simulink model "UberSpurs_oneSpur"  (R2015b)
settings: Solver=VariableStepAuto  StartTime=0.0  StopTime=5000  RelTol=1e-3
libraries: simulink x18
(part 2 of 2)

== system UberSpurs_oneSpur/spur1WorkCell/route2Channel2 ==
  serverAvailable : Inport
  Constant : Constant  Value=2
  Get Attribute : GetAttribute  AttributeName=Channel  EvaluatedDefaultAttributeValue={ []}
      settings: OutputPortMap=o1
  RoutingControlActuator : OutputSwitch  NumberOutputPorts=2  SwitchingCriterion=From signal port p  InitialConditionsOpt=on
  RoutingControlBehavior : Stateflow chart  TreatAsAtomicUnit=on
  Single Server1 : SingleServer  ServiceTime=0
  toChannel : PMIOPort  Port=1  Side=Right
  fromMHS : PMIOPort  Port=2  Side=Left
  toMHS : PMIOPort  Port=3  Side=Right
  wires:
  RoutingControlBehavior/1(route) -> RoutingControlActuator/1
  Constant/1 -> RoutingControlBehavior/2(channel)
  Get Attribute/1 -> RoutingControlBehavior/1(entityChannel)
  serverAvailable/1 -> RoutingControlBehavior/3(serverAvailable)
  connections:
  RoutingControlActuator/RConn2 -- toMHS/RConn1
  Get Attribute/RConn1 -- Single Server1/LConn1
  fromMHS/RConn1 -- Get Attribute/LConn1
  toChannel/RConn1 -- RoutingControlActuator/RConn1
  Single Server1/RConn1 -- RoutingControlActuator/LConn1

== system UberSpurs_oneSpur/spur1WorkCell/route2Channel3 ==
  serverAvailable : Inport
  Constant : Constant  Value=3
  Get Attribute : GetAttribute  AttributeName=Channel  EvaluatedDefaultAttributeValue={ []}
      settings: OutputPortMap=o1
  RoutingControlActuator : OutputSwitch  NumberOutputPorts=2  SwitchingCriterion=From signal port p  InitialConditionsOpt=on
  RoutingControlBehavior : Stateflow chart  TreatAsAtomicUnit=on
  Single Server1 : SingleServer  ServiceTime=0
  toChannel : PMIOPort  Port=1  Side=Right
  fromMHS : PMIOPort  Port=2  Side=Left
  toMHS : PMIOPort  Port=3  Side=Right
  wires:
  RoutingControlBehavior/1(route) -> RoutingControlActuator/1
  Constant/1 -> RoutingControlBehavior/2(channel)
  Get Attribute/1 -> RoutingControlBehavior/1(entityChannel)
  serverAvailable/1 -> RoutingControlBehavior/3(serverAvailable)
  connections:
  RoutingControlActuator/RConn2 -- toMHS/RConn1
  Get Attribute/RConn1 -- Single Server1/LConn1
  fromMHS/RConn1 -- Get Attribute/LConn1
  toChannel/RConn1 -- RoutingControlActuator/RConn1
  Single Server1/RConn1 -- RoutingControlActuator/LConn1

== system UberSpurs_oneSpur/spur1WorkCell/route2Channel4 ==
  serverAvailable : Inport
  Constant : Constant  Value=4
  Get Attribute : GetAttribute  AttributeName=Channel  EvaluatedDefaultAttributeValue={ []}
      settings: OutputPortMap=o1
  RoutingControlActuator : OutputSwitch  NumberOutputPorts=2  SwitchingCriterion=From signal port p  InitialConditionsOpt=on
  RoutingControlBehavior : Stateflow chart  TreatAsAtomicUnit=on
  Single Server1 : SingleServer  ServiceTime=0
  toChannel : PMIOPort  Port=1  Side=Right
  fromMHS : PMIOPort  Port=2  Side=Left
  toMHS : PMIOPort  Port=3  Side=Right
  wires:
  RoutingControlBehavior/1(route) -> RoutingControlActuator/1
  Constant/1 -> RoutingControlBehavior/2(channel)
  Get Attribute/1 -> RoutingControlBehavior/1(entityChannel)
  serverAvailable/1 -> RoutingControlBehavior/3(serverAvailable)
  connections:
  RoutingControlActuator/RConn2 -- toMHS/RConn1
  Get Attribute/RConn1 -- Single Server1/LConn1
  fromMHS/RConn1 -- Get Attribute/LConn1
  toChannel/RConn1 -- RoutingControlActuator/RConn1
  Single Server1/RConn1 -- RoutingControlActuator/LConn1

== system UberSpurs_oneSpur/spur1WorkCell/route2Channel5 ==
  serverAvailable : Inport
  Constant : Constant  Value=5
  Get Attribute : GetAttribute  AttributeName=Channel  EvaluatedDefaultAttributeValue={ []}
      settings: OutputPortMap=o1
  RoutingControlActuator : OutputSwitch  NumberOutputPorts=2  SwitchingCriterion=From signal port p  InitialConditionsOpt=on
  RoutingControlBehavior : Stateflow chart  TreatAsAtomicUnit=on
  Single Server1 : SingleServer  ServiceTime=0
  toChannel : PMIOPort  Port=1  Side=Right
  fromMHS : PMIOPort  Port=2  Side=Left
  toMHS : PMIOPort  Port=3  Side=Right
  wires:
  RoutingControlBehavior/1(route) -> RoutingControlActuator/1
  Constant/1 -> RoutingControlBehavior/2(channel)
  Get Attribute/1 -> RoutingControlBehavior/1(entityChannel)
  serverAvailable/1 -> RoutingControlBehavior/3(serverAvailable)
  connections:
  RoutingControlActuator/RConn2 -- toMHS/RConn1
  Get Attribute/RConn1 -- Single Server1/LConn1
  fromMHS/RConn1 -- Get Attribute/LConn1
  toChannel/RConn1 -- RoutingControlActuator/RConn1
  Single Server1/RConn1 -- RoutingControlActuator/LConn1

== system UberSpurs_oneSpur/spur1WorkCell/route2Channel6 ==
  serverAvailable : Inport
  Constant : Constant  Value=6
  Get Attribute : GetAttribute  AttributeName=Channel  EvaluatedDefaultAttributeValue={ []}
      settings: OutputPortMap=o1
  RoutingControlActuator : OutputSwitch  NumberOutputPorts=2  SwitchingCriterion=From signal port p  InitialConditionsOpt=on
  RoutingControlBehavior : Stateflow chart  TreatAsAtomicUnit=on
  Single Server1 : SingleServer  ServiceTime=0
  toChannel : PMIOPort  Port=1  Side=Right
  fromMHS : PMIOPort  Port=2  Side=Left
  toMHS : PMIOPort  Port=3  Side=Right
  wires:
  RoutingControlBehavior/1(route) -> RoutingControlActuator/1
  Constant/1 -> RoutingControlBehavior/2(channel)
  Get Attribute/1 -> RoutingControlBehavior/1(entityChannel)
  serverAvailable/1 -> RoutingControlBehavior/3(serverAvailable)
  connections:
  RoutingControlActuator/RConn2 -- toMHS/RConn1
  Get Attribute/RConn1 -- Single Server1/LConn1
  fromMHS/RConn1 -- Get Attribute/LConn1
  toChannel/RConn1 -- RoutingControlActuator/RConn1
  Single Server1/RConn1 -- RoutingControlActuator/LConn1

== system UberSpurs_oneSpur/spur1WorkCell/route2Channel7 ==
  serverAvailable : Inport
  Constant : Constant  Value=7
  Get Attribute : GetAttribute  AttributeName=Channel  EvaluatedDefaultAttributeValue={ []}
      settings: OutputPortMap=o1
  RoutingControlActuator : OutputSwitch  NumberOutputPorts=2  SwitchingCriterion=From signal port p  InitialConditionsOpt=on
  RoutingControlBehavior : Stateflow chart  TreatAsAtomicUnit=on
  Single Server1 : SingleServer  ServiceTime=0
  toChannel : PMIOPort  Port=1  Side=Right
  fromMHS : PMIOPort  Port=2  Side=Left
  toMHS : PMIOPort  Port=3  Side=Right
  wires:
  RoutingControlBehavior/1(route) -> RoutingControlActuator/1
  Constant/1 -> RoutingControlBehavior/2(channel)
  Get Attribute/1 -> RoutingControlBehavior/1(entityChannel)
  serverAvailable/1 -> RoutingControlBehavior/3(serverAvailable)
  connections:
  RoutingControlActuator/RConn2 -- toMHS/RConn1
  Get Attribute/RConn1 -- Single Server1/LConn1
  fromMHS/RConn1 -- Get Attribute/LConn1
  toChannel/RConn1 -- RoutingControlActuator/RConn1
  Single Server1/RConn1 -- RoutingControlActuator/LConn1

== system UberSpurs_oneSpur/spur1WorkCell/route2Channel8 ==
  serverAvailable : Inport
  Constant : Constant  Value=8
  Get Attribute : GetAttribute  AttributeName=Channel  EvaluatedDefaultAttributeValue={ []}
      settings: OutputPortMap=o1
  RoutingControlActuator : OutputSwitch  NumberOutputPorts=2  SwitchingCriterion=From signal port p  InitialConditionsOpt=on
  RoutingControlBehavior : Stateflow chart  TreatAsAtomicUnit=on
  Single Server1 : SingleServer  ServiceTime=0
  toChannel : PMIOPort  Port=1  Side=Right
  fromMHS : PMIOPort  Port=2  Side=Left
  toMHS : PMIOPort  Port=3  Side=Right
  wires:
  RoutingControlBehavior/1(route) -> RoutingControlActuator/1
  Constant/1 -> RoutingControlBehavior/2(channel)
  Get Attribute/1 -> RoutingControlBehavior/1(entityChannel)
  serverAvailable/1 -> RoutingControlBehavior/3(serverAvailable)
  connections:
  RoutingControlActuator/RConn2 -- toMHS/RConn1
  Get Attribute/RConn1 -- Single Server1/LConn1
  fromMHS/RConn1 -- Get Attribute/LConn1
  toChannel/RConn1 -- RoutingControlActuator/RConn1
  Single Server1/RConn1 -- RoutingControlActuator/LConn1

== system UberSpurs_oneSpur/spur1WorkCell/route2Channel9 ==
  serverAvailable : Inport
  Constant : Constant  Value=9
  Get Attribute : GetAttribute  AttributeName=Channel  EvaluatedDefaultAttributeValue={ []}
      settings: OutputPortMap=o1
  RoutingControlActuator : OutputSwitch  NumberOutputPorts=2  SwitchingCriterion=From signal port p  InitialConditionsOpt=on
  RoutingControlBehavior : Stateflow chart  TreatAsAtomicUnit=on
  Single Server1 : SingleServer  ServiceTime=0
  toChannel : PMIOPort  Port=1  Side=Right
  fromMHS : PMIOPort  Port=2  Side=Left
  toMHS : PMIOPort  Port=3  Side=Right
  wires:
  RoutingControlBehavior/1(route) -> RoutingControlActuator/1
  Constant/1 -> RoutingControlBehavior/2(channel)
  Get Attribute/1 -> RoutingControlBehavior/1(entityChannel)
  serverAvailable/1 -> RoutingControlBehavior/3(serverAvailable)
  connections:
  RoutingControlActuator/RConn2 -- toMHS/RConn1
  Get Attribute/RConn1 -- Single Server1/LConn1
  fromMHS/RConn1 -- Get Attribute/LConn1
  toChannel/RConn1 -- RoutingControlActuator/RConn1
  Single Server1/RConn1 -- RoutingControlActuator/LConn1

== system UberSpurs_oneSpur/spur1WorkCell/route2recirculate ==
  verifyQueueLength : Inport
  Chart : Stateflow chart  TreatAsAtomicUnit=on
  Get Attribute : GetAttribute  AttributeName=FillTime  EvaluatedDefaultAttributeValue={ []}
      settings: OutputPortMap=o1
  Single Server1 : SingleServer  ServiceTime=0
  route2recirculate : OutputSwitch  NumberOutputPorts=2  SwitchingCriterion=From signal port p  InitialConditionsOpt=on  StatNumberDeparted=on  StatLastDeparturePort=on
      settings: OutputPortMap=o0,o3
  recirculate : PMIOPort  Port=1  Side=Right
  fromMHS : PMIOPort  Port=2  Side=Left
  toverify : PMIOPort  Port=3  Side=Right
  wires:
  Chart/1(route) -> route2recirculate/1
  Get Attribute/1 -> Chart/1(FillTime)
  route2recirculate/1 -> ?
  route2recirculate/2 -> ?
  verifyQueueLength/1 -> Chart/2(verifyQueue)
  connections:
  Get Attribute/RConn1 -- Single Server1/LConn1
  fromMHS/RConn1 -- Get Attribute/LConn1
  Single Server1/RConn1 -- route2recirculate/LConn1
  route2recirculate/RConn2 -- toverify/RConn1
  route2recirculate/RConn1 -- recirculate/RConn1

== system UberSpurs_oneSpur/spur1WorkCell/verifyWorkstation ==
  Clock : Clock
  Set Attribute1 : SetAttribute  AttributeName=VerifyTime  AttributeFrom=Signal port  EvaluatedAttributeValue={ []}
  Timed to Event Sigal : TimedToEventSignal
  VerifyQueue : FIFOQueue  Capacity=1  StatNumberInBlock=on
      settings: OutputPortMap=o1
  VerifyServer : SingleServer  ServiceTimeFrom=Signal port t  ServiceTime=1.55
  processTime : EventBasedRandomNumber  Distribution=Arbitrary discrete  valueVecDisc=[0 1.45]  probVecDisc=[0 1]  Seed=19165
  vialOUT : PMIOPort  Port=1  Side=Left
  vialIN : PMIOPort  Port=2  Side=Right
  queueLength : Outport
  wires:
  processTime/1 -> VerifyServer/1
  Clock/1 -> Timed to Event Sigal/1
  Timed to Event Sigal/1 -> Set Attribute1/1
  VerifyQueue/1 -> queueLength/1
  connections:
  Set Attribute1/RConn1 -- vialOUT/RConn1
  VerifyQueue/RConn1 -- VerifyServer/LConn1
  VerifyQueue/LConn1 -- vialIN/RConn1
  Set Attribute1/LConn1 -- VerifyServer/RConn1

== stateflow chart UberSpurs_oneSpur/route2Spur1/routingControl ==
  (default) -> (junction 9) : % route2Spur
  (junction 9) -> (junction 10) [order 1] : [entitySpur == 1]
  (junction 9) -> (junction 11) [order 2] : {route = 1;}
  (junction 10) -> (junction 12) : {route = 2;}
  (junction 12) -> (junction 11)
  (junction 11) -> (junction 13)
  data: entitySpur input; route output

== stateflow chart UberSpurs_oneSpur/spur1WorkCell/route2Channel2/RoutingControlBehavior ==
  (default) -> (junction 7) : % toChanel
  (junction 7) -> (junction 8) [order 1] : [entityChannel == channel && serverAvailable ==1]
  (junction 7) -> (junction 9) [order 2] : {route = 2;}
  (junction 8) -> (junction 10) : {route = 1 ;}
  (junction 10) -> (junction 9)
  (junction 9) -> (junction 11)
  data: entityChannel input; channel input; route output; serverAvailable input

== stateflow chart UberSpurs_oneSpur/spur1WorkCell/route2Channel1/RoutingControlBehavior ==
  (default) -> (junction 7) : % toChanel
  (junction 7) -> (junction 8) [order 1] : [entityChannel == channel && serverAvailable ==1]
  (junction 7) -> (junction 9) [order 2] : {route = 2;}
  (junction 8) -> (junction 10) : {route = 1 ;}
  (junction 10) -> (junction 9)
  (junction 9) -> (junction 11)
  data: entityChannel input; channel input; route output; serverAvailable input

== stateflow chart UberSpurs_oneSpur/spur1WorkCell/route2Channel3/RoutingControlBehavior ==
  (default) -> (junction 7) : % toChanel
  (junction 7) -> (junction 8) [order 1] : [entityChannel == channel && serverAvailable ==1]
  (junction 7) -> (junction 9) [order 2] : {route = 2;}
  (junction 8) -> (junction 10) : {route = 1 ;}
  (junction 10) -> (junction 9)
  (junction 9) -> (junction 11)
  data: entityChannel input; channel input; route output; serverAvailable input

== stateflow chart UberSpurs_oneSpur/spur1WorkCell/route2Channel4/RoutingControlBehavior ==
  (default) -> (junction 7) : % toChanel
  (junction 7) -> (junction 8) [order 1] : [entityChannel == channel && serverAvailable ==1]
  (junction 7) -> (junction 9) [order 2] : {route = 2;}
  (junction 8) -> (junction 10) : {route = 1 ;}
  (junction 10) -> (junction 9)
  (junction 9) -> (junction 11)
  data: entityChannel input; channel input; route output; serverAvailable input

== stateflow chart UberSpurs_oneSpur/spur1WorkCell/route2Channel5/RoutingControlBehavior ==
  (default) -> (junction 7) : % toChanel
  (junction 7) -> (junction 8) [order 1] : [entityChannel == channel && serverAvailable ==1]
  (junction 7) -> (junction 9) [order 2] : {route = 2;}
  (junction 8) -> (junction 10) : {route = 1 ;}
  (junction 10) -> (junction 9)
  (junction 9) -> (junction 11)
  data: entityChannel input; channel input; route output; serverAvailable input

== stateflow chart UberSpurs_oneSpur/spur1WorkCell/route2Channel6/RoutingControlBehavior ==
  (default) -> (junction 7) : % toChanel
  (junction 7) -> (junction 8) [order 1] : [entityChannel == channel && serverAvailable ==1]
  (junction 7) -> (junction 9) [order 2] : {route = 2;}
  (junction 8) -> (junction 10) : {route = 1 ;}
  (junction 10) -> (junction 9)
  (junction 9) -> (junction 11)
  data: entityChannel input; channel input; route output; serverAvailable input

== stateflow chart UberSpurs_oneSpur/spur1WorkCell/route2Channel7/RoutingControlBehavior ==
  (default) -> (junction 7) : % toChanel
  (junction 7) -> (junction 8) [order 1] : [entityChannel == channel && serverAvailable ==1]
  (junction 7) -> (junction 9) [order 2] : {route = 2;}
  (junction 8) -> (junction 10) : {route = 1 ;}
  (junction 10) -> (junction 9)
  (junction 9) -> (junction 11)
  data: entityChannel input; channel input; route output; serverAvailable input

== stateflow chart UberSpurs_oneSpur/spur1WorkCell/route2Channel8/RoutingControlBehavior ==
  (default) -> (junction 7) : % toChanel
  (junction 7) -> (junction 8) [order 1] : [entityChannel == channel && serverAvailable ==1]
  (junction 7) -> (junction 9) [order 2] : {route = 2;}
  (junction 8) -> (junction 10) : {route = 1 ;}
  (junction 10) -> (junction 9)
  (junction 9) -> (junction 11)
  data: entityChannel input; channel input; route output; serverAvailable input

== stateflow chart UberSpurs_oneSpur/spur1WorkCell/route2Channel9/RoutingControlBehavior ==
  (default) -> (junction 7) : % toChanel
  (junction 7) -> (junction 8) [order 1] : [entityChannel == channel && serverAvailable ==1]
  (junction 7) -> (junction 9) [order 2] : {route = 2;}
  (junction 8) -> (junction 10) : {route = 1 ;}
  (junction 10) -> (junction 9)
  (junction 9) -> (junction 11)
  data: entityChannel input; channel input; route output; serverAvailable input

== stateflow chart UberSpurs_oneSpur/spur1WorkCell/route2recirculate/Chart ==
  (default) -> (junction 7) : % recirculate
  (junction 7) -> (junction 9) [order 1] : [FillTime>0]
  (junction 9) -> (junction 23) [order 1] : [verifyQueue<1]
  (junction 9) -> (junction 20) [order 2] : {route = 1;}
  (junction 7) -> (junction 8) [order 2] : {route = 1;}
  (junction 23) -> (junction 25) : {route = 2;}
  (junction 20) -> (junction 8)
  (junction 25) -> (junction 20)
  (junction 8) -> (junction 11)
  data: FillTime input; route output; verifyQueue input

== stateflow chart UberSpurs_oneSpur/AdmissionControlBehavior ==
  (default) -> (junction 7) : % wipLimit
  (junction 7) -> (junction 8) [order 1] : [WIP <= 64]
  (junction 7) -> (junction 9) [order 2] : {admission = 0;}
  (junction 8) -> (junction 10) : {admission = 1;}
  (junction 10) -> (junction 9)
  (junction 9) -> (junction 11)
  data: WIP input; admission output

== stateflow chart UberSpurs_oneSpur/spur1WorkCell/route2Channel10/RoutingControlBehavior ==
  (default) -> (junction 7) : % toChanel
  (junction 7) -> (junction 8) [order 1] : [entityChannel == channel && serverAvailable ==1]
  (junction 7) -> (junction 9) [order 2] : {route = 2;}
  (junction 8) -> (junction 10) : {route = 1 ;}
  (junction 10) -> (junction 9)
  (junction 9) -> (junction 11)
  data: entityChannel input; channel input; route output; serverAvailable input

== stateflow chart UberSpurs_oneSpur/spur1WorkCell/route2Channel11/RoutingControlBehavior ==
  (default) -> (junction 7) : % toChanel
  (junction 7) -> (junction 8) [order 1] : [entityChannel == channel && serverAvailable ==1]
  (junction 7) -> (junction 9) [order 2] : {route = 2;}
  (junction 8) -> (junction 10) : {route = 1 ;}
  (junction 10) -> (junction 9)
  (junction 9) -> (junction 11)
  data: entityChannel input; channel input; route output; serverAvailable input

== stateflow chart UberSpurs_oneSpur/spur1WorkCell/route2Channel12/RoutingControlBehavior ==
  (default) -> (junction 7) : % toChanel
  (junction 7) -> (junction 8) [order 1] : [entityChannel == channel && serverAvailable ==1]
  (junction 7) -> (junction 9) [order 2] : {route = 2;}
  (junction 8) -> (junction 10) : {route = 1 ;}
  (junction 10) -> (junction 9)
  (junction 9) -> (junction 11)
  data: entityChannel input; channel input; route output; serverAvailable input

== stateflow chart UberSpurs_oneSpur/spur1WorkCell/route2Channel13/RoutingControlBehavior ==
  (default) -> (junction 7) : % toChanel
  (junction 7) -> (junction 8) [order 1] : [entityChannel == channel && serverAvailable ==1]
  (junction 7) -> (junction 9) [order 2] : {route = 2;}
  (junction 8) -> (junction 10) : {route = 1 ;}
  (junction 10) -> (junction 9)
  (junction 9) -> (junction 11)
  data: entityChannel input; channel input; route output; serverAvailable input

== stateflow chart UberSpurs_oneSpur/spur1WorkCell/route2Channel14/RoutingControlBehavior ==
  (default) -> (junction 7) : % toChanel
  (junction 7) -> (junction 8) [order 1] : [entityChannel == channel && serverAvailable ==1]
  (junction 7) -> (junction 9) [order 2] : {route = 2;}
  (junction 8) -> (junction 10) : {route = 1 ;}
  (junction 10) -> (junction 9)
  (junction 9) -> (junction 11)
  data: entityChannel input; channel input; route output; serverAvailable input

== stateflow chart UberSpurs_oneSpur/spur1WorkCell/route2Channel15/RoutingControlBehavior ==
  (default) -> (junction 7) : % toChanel
  (junction 7) -> (junction 8) [order 1] : [entityChannel == channel && serverAvailable ==1]
  (junction 7) -> (junction 9) [order 2] : {route = 2;}
  (junction 8) -> (junction 10) : {route = 1 ;}
  (junction 10) -> (junction 9)
  (junction 9) -> (junction 11)
  data: entityChannel input; channel input; route output; serverAvailable input

== stateflow chart UberSpurs_oneSpur/spur1WorkCell/route2Channel16/RoutingControlBehavior ==
  (default) -> (junction 7) : % toChanel
  (junction 7) -> (junction 8) [order 1] : [entityChannel == channel && serverAvailable ==1]
  (junction 7) -> (junction 9) [order 2] : {route = 2;}
  (junction 8) -> (junction 10) : {route = 1 ;}
  (junction 10) -> (junction 9)
  (junction 9) -> (junction 11)
  data: entityChannel input; channel input; route output; serverAvailable input

== stateflow chart UberSpurs_oneSpur/spur1WorkCell/route2Channel17/RoutingControlBehavior ==
  (default) -> (junction 7) : % toChanel
  (junction 7) -> (junction 8) [order 1] : [entityChannel == channel && serverAvailable ==1]
  (junction 7) -> (junction 9) [order 2] : {route = 2;}
  (junction 8) -> (junction 10) : {route = 1 ;}
  (junction 10) -> (junction 9)
  (junction 9) -> (junction 11)
  data: entityChannel input; channel input; route output; serverAvailable input

== stateflow chart UberSpurs_oneSpur/spur1WorkCell/route2Channel18/RoutingControlBehavior ==
  (default) -> (junction 7) : % toChanel
  (junction 7) -> (junction 8) [order 1] : [entityChannel == channel && serverAvailable ==1]
  (junction 7) -> (junction 9) [order 2] : {route = 2;}
  (junction 8) -> (junction 10) : {route = 1 ;}
  (junction 10) -> (junction 9)
  (junction 9) -> (junction 11)
  data: entityChannel input; channel input; route output; serverAvailable input
